simulink model "wheel_model"  (R2016a)
settings: Solver=VariableStepAuto  StartTime=0.0  StopTime=10.0  RelTol=1e-3
undefined symbols (not defined in the file): Iw, r
settings Model: Creator=mgreiff  LastModifiedBy=mgreiff

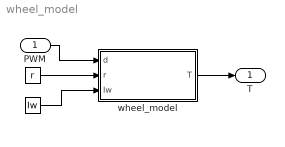
== system wheel_model ==
  PWM : Inport
  " " : Constant  Value=r
  "  " : Constant  Value=Iw
  wheel_model : MATLAB Function  TreatAsAtomicUnit=on
  T : Outport  PortDimensions=3
  wires:
  PWM/1 -> wheel_model/1(d)
  " "/1 -> wheel_model/2(r)
  "  "/1 -> wheel_model/3(Iw)
  wheel_model/1(T) -> T/1

== matlab function wheel_model/wheel_model ==
  data: d input; T output; r input; Iw input
function T = wheel_model(d, r, Iw)
%#codegen

% Todo find map from d -> ddtheta
ddtheta = d;
T = [ddtheta * ( Iw / r );0;0];
